simulink model "FINAL"  (R2019a)
settings: Solver=VariableStepAuto  StartTime=0.0  StopTime=5  FixedStep=0.0001  RelTol=1e-3
PreLoadFcn:
  | initDuckWPT
InitFcn:
  | initDuckWPT
StartFcn:
  | initDuckWPT
values from neighbouring files (symbols this model uses):
  angleTolerance = 2    [initDuckWPT.m]
  eeTolerance = 0.01    [initDuckWPT.m]
  JointBounds1 = [-pi/2       pi ... (first row only)    [initDuckWPT.m]
  JointBounds2 = [-pi/3       pi/3 ... (first row only)    [initDuckWPT.m]
  rotM1 = roty(90)*rotx(90)    [initDuckWPT.m]
  trajectory = [0.4  0.4  0.4  0.4  0.4  0.4  0.4 ... (first row only)    [initDuckWPT.m]
undefined symbols (not defined in the file or in its folder): DiscIntNeverNeededParam, X, Y, Z
libraries: sm_lib x205, fl_lib x72, nesl_utility x43, fl_ps_legacy_lib x18, fuzblock x16, Contact_Forces_Lib x12
(part 7 of 7)

== system FINAL/Environment/Robot/Rotational Hardstop51/  1 ==
  External Force and Torque B : sm_lib/Forces and Torques/External Force and Torque  ForceResolutionFrame=AttachedFrame  EnableForceX=off  EnableForceY=off  EnableForceZ=off  EnableForce=off  TorqueResolutionFrame=AttachedFrame  EnableTorqueX=off  EnableTorqueY=off  EnableTorqueZ=on  EnableTorque=off
  External Force and Torque F : sm_lib/Forces and Torques/External Force and Torque  ForceResolutionFrame=AttachedFrame  EnableForceX=off  EnableForceY=off  EnableForceZ=off  EnableForce=off  TorqueResolutionFrame=AttachedFrame  EnableTorqueX=off  EnableTorqueY=off  EnableTorqueZ=on  EnableTorque=off
  Ideal Angular Velocity Source : fl_lib/Mechanical/Mechanical Sources/Ideal Angular Velocity Source
  Ideal Torque Sensor : fl_lib/Mechanical/Mechanical Sensors/Ideal Torque Sensor
  Sign Force B : fl_ps_legacy_lib/Legacy Physical Signals/Functions/PS Gain  gain=-1
      settings: SourceProductName=Simscape
  Transform Sensor : sm_lib/Frames and Transforms/Transform Sensor  MeasurementFrame=Base  SenseAngle=off  SenseAxis=off  SenseAngle1=off  SenseAngle2=off  SenseAngle3=off  SenseQ=off  SenseR=off  SenseOmegaX=off  SenseOmegaY=off  SenseOmegaZ=on  SenseOmega1=off  SenseOmega2=off  SenseOmega3=off  SenseQDot=off  SenseRDot=off  SenseAlphaX=off  SenseAlphaY=off  SenseAlphaZ=off  SenseAlpha1=off  SenseAlpha2=off  SenseAlpha3=off  SenseQDDot=off  SenseRDDot=off  SenseX=off  SenseY=off  SenseZ=off  SenseRad=off  SenseAzim=off  SenseDist=off  SenseInc=off  SenseXDot=off  SenseYDot=off  SenseZDot=off  SenseRadDot=off  SenseAzimDot=off  SenseDistDot=off  SenseIncDot=off  SenseXDDot=off  SenseYDDot=off  SenseZDDot=off  SenseRadDDot=off  SenseAzimDDot=off  SenseDistDDot=off  SenseIncDDot=off
  B : PMIOPort  Side=Left
  F : PMIOPort  Port=2  Side=Right
  R : PMIOPort  Port=3  Side=Right
  C : PMIOPort  Port=4  Side=Left
  connections:
  Ideal Angular Velocity Source/RConn1 -- Transform Sensor/RConn2
  Sign Force B/RConn1 -- External Force and Torque B/LConn1
  B/RConn1 -- External Force and Torque B/RConn1 -- Transform Sensor/LConn1
  External Force and Torque F/RConn1 -- Transform Sensor/RConn1 -- F/RConn1
  C/RConn1 -- Ideal Torque Sensor/RConn1
  External Force and Torque F/LConn1 -- Sign Force B/LConn1 -- Ideal Torque Sensor/RConn2
  Ideal Torque Sensor/LConn1 -- Ideal Angular Velocity Source/RConn2
  R/RConn1 -- Ideal Angular Velocity Source/LConn1

== system FINAL/Environment/Robot/Rotational Hardstop52/  1 ==
  External Force and Torque B : sm_lib/Forces and Torques/External Force and Torque  ForceResolutionFrame=AttachedFrame  EnableForceX=off  EnableForceY=off  EnableForceZ=off  EnableForce=off  TorqueResolutionFrame=AttachedFrame  EnableTorqueX=off  EnableTorqueY=off  EnableTorqueZ=on  EnableTorque=off
  External Force and Torque F : sm_lib/Forces and Torques/External Force and Torque  ForceResolutionFrame=AttachedFrame  EnableForceX=off  EnableForceY=off  EnableForceZ=off  EnableForce=off  TorqueResolutionFrame=AttachedFrame  EnableTorqueX=off  EnableTorqueY=off  EnableTorqueZ=on  EnableTorque=off
  Ideal Angular Velocity Source : fl_lib/Mechanical/Mechanical Sources/Ideal Angular Velocity Source
  Ideal Torque Sensor : fl_lib/Mechanical/Mechanical Sensors/Ideal Torque Sensor
  Sign Force B : fl_ps_legacy_lib/Legacy Physical Signals/Functions/PS Gain  gain=-1
      settings: SourceProductName=Simscape
  Transform Sensor : sm_lib/Frames and Transforms/Transform Sensor  MeasurementFrame=Base  SenseAngle=off  SenseAxis=off  SenseAngle1=off  SenseAngle2=off  SenseAngle3=off  SenseQ=off  SenseR=off  SenseOmegaX=off  SenseOmegaY=off  SenseOmegaZ=on  SenseOmega1=off  SenseOmega2=off  SenseOmega3=off  SenseQDot=off  SenseRDot=off  SenseAlphaX=off  SenseAlphaY=off  SenseAlphaZ=off  SenseAlpha1=off  SenseAlpha2=off  SenseAlpha3=off  SenseQDDot=off  SenseRDDot=off  SenseX=off  SenseY=off  SenseZ=off  SenseRad=off  SenseAzim=off  SenseDist=off  SenseInc=off  SenseXDot=off  SenseYDot=off  SenseZDot=off  SenseRadDot=off  SenseAzimDot=off  SenseDistDot=off  SenseIncDot=off  SenseXDDot=off  SenseYDDot=off  SenseZDDot=off  SenseRadDDot=off  SenseAzimDDot=off  SenseDistDDot=off  SenseIncDDot=off
  B : PMIOPort  Side=Left
  F : PMIOPort  Port=2  Side=Right
  R : PMIOPort  Port=3  Side=Right
  C : PMIOPort  Port=4  Side=Left
  connections:
  R/RConn1 -- Ideal Angular Velocity Source/LConn1
  Ideal Torque Sensor/LConn1 -- Ideal Angular Velocity Source/RConn2
  Ideal Torque Sensor/RConn2 -- Sign Force B/LConn1 -- External Force and Torque F/LConn1
  C/RConn1 -- Ideal Torque Sensor/RConn1
  F/RConn1 -- Transform Sensor/RConn1 -- External Force and Torque F/RConn1
  Transform Sensor/LConn1 -- External Force and Torque B/RConn1 -- B/RConn1
  Sign Force B/RConn1 -- External Force and Torque B/LConn1
  Ideal Angular Velocity Source/RConn1 -- Transform Sensor/RConn2

== system FINAL/Environment/Robot/Rotational Hardstop61/  1 ==
  External Force and Torque B : sm_lib/Forces and Torques/External Force and Torque  ForceResolutionFrame=AttachedFrame  EnableForceX=off  EnableForceY=off  EnableForceZ=off  EnableForce=off  TorqueResolutionFrame=AttachedFrame  EnableTorqueX=off  EnableTorqueY=off  EnableTorqueZ=on  EnableTorque=off
  External Force and Torque F : sm_lib/Forces and Torques/External Force and Torque  ForceResolutionFrame=AttachedFrame  EnableForceX=off  EnableForceY=off  EnableForceZ=off  EnableForce=off  TorqueResolutionFrame=AttachedFrame  EnableTorqueX=off  EnableTorqueY=off  EnableTorqueZ=on  EnableTorque=off
  Ideal Angular Velocity Source : fl_lib/Mechanical/Mechanical Sources/Ideal Angular Velocity Source
  Ideal Torque Sensor : fl_lib/Mechanical/Mechanical Sensors/Ideal Torque Sensor
  Sign Force B : fl_ps_legacy_lib/Legacy Physical Signals/Functions/PS Gain  gain=-1
      settings: SourceProductName=Simscape
  Transform Sensor : sm_lib/Frames and Transforms/Transform Sensor  MeasurementFrame=Base  SenseAngle=off  SenseAxis=off  SenseAngle1=off  SenseAngle2=off  SenseAngle3=off  SenseQ=off  SenseR=off  SenseOmegaX=off  SenseOmegaY=off  SenseOmegaZ=on  SenseOmega1=off  SenseOmega2=off  SenseOmega3=off  SenseQDot=off  SenseRDot=off  SenseAlphaX=off  SenseAlphaY=off  SenseAlphaZ=off  SenseAlpha1=off  SenseAlpha2=off  SenseAlpha3=off  SenseQDDot=off  SenseRDDot=off  SenseX=off  SenseY=off  SenseZ=off  SenseRad=off  SenseAzim=off  SenseDist=off  SenseInc=off  SenseXDot=off  SenseYDot=off  SenseZDot=off  SenseRadDot=off  SenseAzimDot=off  SenseDistDot=off  SenseIncDot=off  SenseXDDot=off  SenseYDDot=off  SenseZDDot=off  SenseRadDDot=off  SenseAzimDDot=off  SenseDistDDot=off  SenseIncDDot=off
  B : PMIOPort  Side=Left
  F : PMIOPort  Port=2  Side=Right
  R : PMIOPort  Port=3  Side=Right
  C : PMIOPort  Port=4  Side=Left
  connections:
  R/RConn1 -- Ideal Angular Velocity Source/LConn1
  Ideal Torque Sensor/LConn1 -- Ideal Angular Velocity Source/RConn2
  Ideal Torque Sensor/RConn2 -- Sign Force B/LConn1 -- External Force and Torque F/LConn1
  C/RConn1 -- Ideal Torque Sensor/RConn1
  F/RConn1 -- Transform Sensor/RConn1 -- External Force and Torque F/RConn1
  Transform Sensor/LConn1 -- External Force and Torque B/RConn1 -- B/RConn1
  Sign Force B/RConn1 -- External Force and Torque B/LConn1
  Ideal Angular Velocity Source/RConn1 -- Transform Sensor/RConn2

== system FINAL/Environment/Robot/Rotational Hardstop62/  1 ==
  External Force and Torque B : sm_lib/Forces and Torques/External Force and Torque  ForceResolutionFrame=AttachedFrame  EnableForceX=off  EnableForceY=off  EnableForceZ=off  EnableForce=off  TorqueResolutionFrame=AttachedFrame  EnableTorqueX=off  EnableTorqueY=off  EnableTorqueZ=on  EnableTorque=off
  External Force and Torque F : sm_lib/Forces and Torques/External Force and Torque  ForceResolutionFrame=AttachedFrame  EnableForceX=off  EnableForceY=off  EnableForceZ=off  EnableForce=off  TorqueResolutionFrame=AttachedFrame  EnableTorqueX=off  EnableTorqueY=off  EnableTorqueZ=on  EnableTorque=off
  Ideal Angular Velocity Source : fl_lib/Mechanical/Mechanical Sources/Ideal Angular Velocity Source
  Ideal Torque Sensor : fl_lib/Mechanical/Mechanical Sensors/Ideal Torque Sensor
  Sign Force B : fl_ps_legacy_lib/Legacy Physical Signals/Functions/PS Gain  gain=-1
      settings: SourceProductName=Simscape
  Transform Sensor : sm_lib/Frames and Transforms/Transform Sensor  MeasurementFrame=Base  SenseAngle=off  SenseAxis=off  SenseAngle1=off  SenseAngle2=off  SenseAngle3=off  SenseQ=off  SenseR=off  SenseOmegaX=off  SenseOmegaY=off  SenseOmegaZ=on  SenseOmega1=off  SenseOmega2=off  SenseOmega3=off  SenseQDot=off  SenseRDot=off  SenseAlphaX=off  SenseAlphaY=off  SenseAlphaZ=off  SenseAlpha1=off  SenseAlpha2=off  SenseAlpha3=off  SenseQDDot=off  SenseRDDot=off  SenseX=off  SenseY=off  SenseZ=off  SenseRad=off  SenseAzim=off  SenseDist=off  SenseInc=off  SenseXDot=off  SenseYDot=off  SenseZDot=off  SenseRadDot=off  SenseAzimDot=off  SenseDistDot=off  SenseIncDot=off  SenseXDDot=off  SenseYDDot=off  SenseZDDot=off  SenseRadDDot=off  SenseAzimDDot=off  SenseDistDDot=off  SenseIncDDot=off
  B : PMIOPort  Side=Left
  F : PMIOPort  Port=2  Side=Right
  R : PMIOPort  Port=3  Side=Right
  C : PMIOPort  Port=4  Side=Left
  connections:
  Ideal Angular Velocity Source/RConn1 -- Transform Sensor/RConn2
  Sign Force B/RConn1 -- External Force and Torque B/LConn1
  B/RConn1 -- External Force and Torque B/RConn1 -- Transform Sensor/LConn1
  External Force and Torque F/RConn1 -- Transform Sensor/RConn1 -- F/RConn1
  C/RConn1 -- Ideal Torque Sensor/RConn1
  External Force and Torque F/LConn1 -- Sign Force B/LConn1 -- Ideal Torque Sensor/RConn2
  Ideal Torque Sensor/LConn1 -- Ideal Angular Velocity Source/RConn2
  R/RConn1 -- Ideal Angular Velocity Source/LConn1

== system FINAL/Environment/Robot/Rotational Hardstop71/  1 ==
  External Force and Torque B : sm_lib/Forces and Torques/External Force and Torque  ForceResolutionFrame=AttachedFrame  EnableForceX=off  EnableForceY=off  EnableForceZ=off  EnableForce=off  TorqueResolutionFrame=AttachedFrame  EnableTorqueX=off  EnableTorqueY=off  EnableTorqueZ=on  EnableTorque=off
  External Force and Torque F : sm_lib/Forces and Torques/External Force and Torque  ForceResolutionFrame=AttachedFrame  EnableForceX=off  EnableForceY=off  EnableForceZ=off  EnableForce=off  TorqueResolutionFrame=AttachedFrame  EnableTorqueX=off  EnableTorqueY=off  EnableTorqueZ=on  EnableTorque=off
  Ideal Angular Velocity Source : fl_lib/Mechanical/Mechanical Sources/Ideal Angular Velocity Source
  Ideal Torque Sensor : fl_lib/Mechanical/Mechanical Sensors/Ideal Torque Sensor
  Sign Force B : fl_ps_legacy_lib/Legacy Physical Signals/Functions/PS Gain  gain=-1
      settings: SourceProductName=Simscape
  Transform Sensor : sm_lib/Frames and Transforms/Transform Sensor  MeasurementFrame=Base  SenseAngle=off  SenseAxis=off  SenseAngle1=off  SenseAngle2=off  SenseAngle3=off  SenseQ=off  SenseR=off  SenseOmegaX=off  SenseOmegaY=off  SenseOmegaZ=on  SenseOmega1=off  SenseOmega2=off  SenseOmega3=off  SenseQDot=off  SenseRDot=off  SenseAlphaX=off  SenseAlphaY=off  SenseAlphaZ=off  SenseAlpha1=off  SenseAlpha2=off  SenseAlpha3=off  SenseQDDot=off  SenseRDDot=off  SenseX=off  SenseY=off  SenseZ=off  SenseRad=off  SenseAzim=off  SenseDist=off  SenseInc=off  SenseXDot=off  SenseYDot=off  SenseZDot=off  SenseRadDot=off  SenseAzimDot=off  SenseDistDot=off  SenseIncDot=off  SenseXDDot=off  SenseYDDot=off  SenseZDDot=off  SenseRadDDot=off  SenseAzimDDot=off  SenseDistDDot=off  SenseIncDDot=off
  B : PMIOPort  Side=Left
  F : PMIOPort  Port=2  Side=Right
  R : PMIOPort  Port=3  Side=Right
  C : PMIOPort  Port=4  Side=Left
  connections:
  Ideal Angular Velocity Source/RConn1 -- Transform Sensor/RConn2
  Sign Force B/RConn1 -- External Force and Torque B/LConn1
  B/RConn1 -- External Force and Torque B/RConn1 -- Transform Sensor/LConn1
  External Force and Torque F/RConn1 -- Transform Sensor/RConn1 -- F/RConn1
  C/RConn1 -- Ideal Torque Sensor/RConn1
  External Force and Torque F/LConn1 -- Sign Force B/LConn1 -- Ideal Torque Sensor/RConn2
  Ideal Torque Sensor/LConn1 -- Ideal Angular Velocity Source/RConn2
  R/RConn1 -- Ideal Angular Velocity Source/LConn1

== system FINAL/Environment/Robot/Rotational Hardstop72/  1 ==
  External Force and Torque B : sm_lib/Forces and Torques/External Force and Torque  ForceResolutionFrame=AttachedFrame  EnableForceX=off  EnableForceY=off  EnableForceZ=off  EnableForce=off  TorqueResolutionFrame=AttachedFrame  EnableTorqueX=off  EnableTorqueY=off  EnableTorqueZ=on  EnableTorque=off
  External Force and Torque F : sm_lib/Forces and Torques/External Force and Torque  ForceResolutionFrame=AttachedFrame  EnableForceX=off  EnableForceY=off  EnableForceZ=off  EnableForce=off  TorqueResolutionFrame=AttachedFrame  EnableTorqueX=off  EnableTorqueY=off  EnableTorqueZ=on  EnableTorque=off
  Ideal Angular Velocity Source : fl_lib/Mechanical/Mechanical Sources/Ideal Angular Velocity Source
  Ideal Torque Sensor : fl_lib/Mechanical/Mechanical Sensors/Ideal Torque Sensor
  Sign Force B : fl_ps_legacy_lib/Legacy Physical Signals/Functions/PS Gain  gain=-1
      settings: SourceProductName=Simscape
  Transform Sensor : sm_lib/Frames and Transforms/Transform Sensor  MeasurementFrame=Base  SenseAngle=off  SenseAxis=off  SenseAngle1=off  SenseAngle2=off  SenseAngle3=off  SenseQ=off  SenseR=off  SenseOmegaX=off  SenseOmegaY=off  SenseOmegaZ=on  SenseOmega1=off  SenseOmega2=off  SenseOmega3=off  SenseQDot=off  SenseRDot=off  SenseAlphaX=off  SenseAlphaY=off  SenseAlphaZ=off  SenseAlpha1=off  SenseAlpha2=off  SenseAlpha3=off  SenseQDDot=off  SenseRDDot=off  SenseX=off  SenseY=off  SenseZ=off  SenseRad=off  SenseAzim=off  SenseDist=off  SenseInc=off  SenseXDot=off  SenseYDot=off  SenseZDot=off  SenseRadDot=off  SenseAzimDot=off  SenseDistDot=off  SenseIncDot=off  SenseXDDot=off  SenseYDDot=off  SenseZDDot=off  SenseRadDDot=off  SenseAzimDDot=off  SenseDistDDot=off  SenseIncDDot=off
  B : PMIOPort  Side=Left
  F : PMIOPort  Port=2  Side=Right
  R : PMIOPort  Port=3  Side=Right
  C : PMIOPort  Port=4  Side=Left
  connections:
  R/RConn1 -- Ideal Angular Velocity Source/LConn1
  Ideal Torque Sensor/LConn1 -- Ideal Angular Velocity Source/RConn2
  Ideal Torque Sensor/RConn2 -- Sign Force B/LConn1 -- External Force and Torque F/LConn1
  C/RConn1 -- Ideal Torque Sensor/RConn1
  F/RConn1 -- Transform Sensor/RConn1 -- External Force and Torque F/RConn1
  Transform Sensor/LConn1 -- External Force and Torque B/RConn1 -- B/RConn1
  Sign Force B/RConn1 -- External Force and Torque B/LConn1
  Ideal Angular Velocity Source/RConn1 -- Transform Sensor/RConn2

== system FINAL/Physical Controller Fuzzy PID/Fuzzy PID Tuning1/Subsystem1/PID ==
  u : Inport
  Kp : Inport  Port=2
  Kd : Inport  Port=3
  Ki : Inport  Port=4
  Discrete-Time Integrator : DiscreteIntegrator  SampleTime=-1  ICPrevOutput=DiscIntNeverNeededParam  ICPrevScaledInput=DiscIntNeverNeededParam
  Discrete-Time Integrator1 : DiscreteIntegrator  SampleTime=-1  ICPrevOutput=DiscIntNeverNeededParam  ICPrevScaledInput=DiscIntNeverNeededParam
  Gain : Gain  Gain=2
  Product : Product
  Product1 : Product
  Product2 : Product
  Sum : Sum  Inputs=|+-
  Sum1 : Sum  Inputs=+++
  Out1 : Outport
  wires:
  Gain/1 -> Sum1/3, Discrete-Time Integrator1/1
  Kp/1 -> Product/2
  u/1 -> Discrete-Time Integrator/1, Product2/1, Product/1
  Kd/1 -> Product2/2
  Product2/1 -> Sum/1
  Discrete-Time Integrator1/1 -> Sum/2
  Sum/1 -> Gain/1
  Product/1 -> Sum1/1
  Sum1/1 -> Out1/1
  Ki/1 -> Product1/2
  Discrete-Time Integrator/1 -> Product1/1
  Product1/1 -> Sum1/2

== system FINAL/Physical Controller Fuzzy PID/Fuzzy PID Tuning1/Subsystem2/PID ==
  u : Inport
  Kp : Inport  Port=2
  Kd : Inport  Port=3
  Ki : Inport  Port=4
  Discrete-Time Integrator : DiscreteIntegrator  SampleTime=-1  ICPrevOutput=DiscIntNeverNeededParam  ICPrevScaledInput=DiscIntNeverNeededParam
  Discrete-Time Integrator1 : DiscreteIntegrator  SampleTime=-1  ICPrevOutput=DiscIntNeverNeededParam  ICPrevScaledInput=DiscIntNeverNeededParam
  Gain : Gain  Gain=2
  Product : Product
  Product1 : Product
  Product2 : Product
  Sum : Sum  Inputs=|+-
  Sum1 : Sum  Inputs=+++
  Out1 : Outport
  wires:
  Product1/1 -> Sum1/2
  Discrete-Time Integrator/1 -> Product1/1
  Ki/1 -> Product1/2
  Sum1/1 -> Out1/1
  Product/1 -> Sum1/1
  Sum/1 -> Gain/1
  Discrete-Time Integrator1/1 -> Sum/2
  Product2/1 -> Sum/1
  Kd/1 -> Product2/2
  u/1 -> Product/1, Product2/1, Discrete-Time Integrator/1
  Kp/1 -> Product/2
  Gain/1 -> Discrete-Time Integrator1/1, Sum1/3

== system FINAL/Physical Controller Fuzzy PID/Fuzzy PID Tuning1/Subsystem3/PID ==
  u : Inport
  Kp : Inport  Port=2
  Kd : Inport  Port=3
  Ki : Inport  Port=4
  Discrete-Time Integrator : DiscreteIntegrator  SampleTime=-1  ICPrevOutput=DiscIntNeverNeededParam  ICPrevScaledInput=DiscIntNeverNeededParam
  Discrete-Time Integrator1 : DiscreteIntegrator  SampleTime=-1  ICPrevOutput=DiscIntNeverNeededParam  ICPrevScaledInput=DiscIntNeverNeededParam
  Gain : Gain  Gain=2
  Product : Product
  Product1 : Product
  Product2 : Product
  Sum : Sum  Inputs=|+-
  Sum1 : Sum  Inputs=+++
  Out1 : Outport
  wires:
  Product1/1 -> Sum1/2
  Discrete-Time Integrator/1 -> Product1/1
  Ki/1 -> Product1/2
  Sum1/1 -> Out1/1
  Product/1 -> Sum1/1
  Sum/1 -> Gain/1
  Discrete-Time Integrator1/1 -> Sum/2
  Product2/1 -> Sum/1
  Kd/1 -> Product2/2
  u/1 -> Product/1, Product2/1, Discrete-Time Integrator/1
  Kp/1 -> Product/2
  Gain/1 -> Discrete-Time Integrator1/1, Sum1/3

== system FINAL/Physical Controller Fuzzy PID/Fuzzy PID Tuning1/Subsystem4/PID ==
  u : Inport
  Kp : Inport  Port=2
  Kd : Inport  Port=3
  Ki : Inport  Port=4
  Discrete-Time Integrator : DiscreteIntegrator  SampleTime=-1  ICPrevOutput=DiscIntNeverNeededParam  ICPrevScaledInput=DiscIntNeverNeededParam
  Discrete-Time Integrator1 : DiscreteIntegrator  SampleTime=-1  ICPrevOutput=DiscIntNeverNeededParam  ICPrevScaledInput=DiscIntNeverNeededParam
  Gain : Gain  Gain=2
  Product : Product
  Product1 : Product
  Product2 : Product
  Sum : Sum  Inputs=|+-
  Sum1 : Sum  Inputs=+++
  Out1 : Outport
  wires:
  Gain/1 -> Sum1/3, Discrete-Time Integrator1/1
  Kp/1 -> Product/2
  u/1 -> Discrete-Time Integrator/1, Product2/1, Product/1
  Kd/1 -> Product2/2
  Product2/1 -> Sum/1
  Discrete-Time Integrator1/1 -> Sum/2
  Sum/1 -> Gain/1
  Product/1 -> Sum1/1
  Sum1/1 -> Out1/1
  Ki/1 -> Product1/2
  Discrete-Time Integrator/1 -> Product1/1
  Product1/1 -> Sum1/2

== system FINAL/Physical Controller Fuzzy PID/Fuzzy PID Tuning1/Subsystem5/PID ==
  u : Inport
  Kp : Inport  Port=2
  Kd : Inport  Port=3
  Ki : Inport  Port=4
  Discrete-Time Integrator : DiscreteIntegrator  SampleTime=-1  ICPrevOutput=DiscIntNeverNeededParam  ICPrevScaledInput=DiscIntNeverNeededParam
  Discrete-Time Integrator1 : DiscreteIntegrator  SampleTime=-1  ICPrevOutput=DiscIntNeverNeededParam  ICPrevScaledInput=DiscIntNeverNeededParam
  Gain : Gain  Gain=2
  Product : Product
  Product1 : Product
  Product2 : Product
  Sum : Sum  Inputs=|+-
  Sum1 : Sum  Inputs=+++
  Out1 : Outport
  wires:
  Product1/1 -> Sum1/2
  Discrete-Time Integrator/1 -> Product1/1
  Ki/1 -> Product1/2
  Sum1/1 -> Out1/1
  Product/1 -> Sum1/1
  Sum/1 -> Gain/1
  Discrete-Time Integrator1/1 -> Sum/2
  Product2/1 -> Sum/1
  Kd/1 -> Product2/2
  u/1 -> Product/1, Product2/1, Discrete-Time Integrator/1
  Kp/1 -> Product/2
  Gain/1 -> Discrete-Time Integrator1/1, Sum1/3

== system FINAL/Physical Controller Fuzzy PID/Fuzzy PID Tuning1/Subsystem6/PID ==
  u : Inport
  Kp : Inport  Port=2
  Kd : Inport  Port=3
  Ki : Inport  Port=4
  Discrete-Time Integrator : DiscreteIntegrator  SampleTime=-1  ICPrevOutput=DiscIntNeverNeededParam  ICPrevScaledInput=DiscIntNeverNeededParam
  Discrete-Time Integrator1 : DiscreteIntegrator  SampleTime=-1  ICPrevOutput=DiscIntNeverNeededParam  ICPrevScaledInput=DiscIntNeverNeededParam
  Gain : Gain  Gain=2
  Product : Product
  Product1 : Product
  Product2 : Product
  Sum : Sum  Inputs=|+-
  Sum1 : Sum  Inputs=+++
  Out1 : Outport
  wires:
  Gain/1 -> Sum1/3, Discrete-Time Integrator1/1
  Kp/1 -> Product/2
  u/1 -> Discrete-Time Integrator/1, Product2/1, Product/1
  Kd/1 -> Product2/2
  Product2/1 -> Sum/1
  Discrete-Time Integrator1/1 -> Sum/2
  Sum/1 -> Gain/1
  Product/1 -> Sum1/1
  Sum1/1 -> Out1/1
  Ki/1 -> Product1/2
  Discrete-Time Integrator/1 -> Product1/1
  Product1/1 -> Sum1/2

== system FINAL/Physical Controller Fuzzy PID/Fuzzy PID Tuning1/Subsystem7/PID ==
  u : Inport
  Kp : Inport  Port=2
  Kd : Inport  Port=3
  Ki : Inport  Port=4
  Discrete-Time Integrator : DiscreteIntegrator  SampleTime=-1  ICPrevOutput=DiscIntNeverNeededParam  ICPrevScaledInput=DiscIntNeverNeededParam
  Discrete-Time Integrator1 : DiscreteIntegrator  SampleTime=-1  ICPrevOutput=DiscIntNeverNeededParam  ICPrevScaledInput=DiscIntNeverNeededParam
  Gain : Gain  Gain=2
  Product : Product
  Product1 : Product
  Product2 : Product
  Sum : Sum  Inputs=|+-
  Sum1 : Sum  Inputs=+++
  Out1 : Outport
  wires:
  Gain/1 -> Sum1/3, Discrete-Time Integrator1/1
  Kp/1 -> Product/2
  u/1 -> Discrete-Time Integrator/1, Product2/1, Product/1
  Kd/1 -> Product2/2
  Product2/1 -> Sum/1
  Discrete-Time Integrator1/1 -> Sum/2
  Sum/1 -> Gain/1
  Product/1 -> Sum1/1
  Sum1/1 -> Out1/1
  Ki/1 -> Product1/2
  Discrete-Time Integrator/1 -> Product1/1
  Product1/1 -> Sum1/2

== system FINAL/Physical Controller Fuzzy PID/Fuzzy PID Tuning1/Subsystem8/PID ==
  u : Inport
  Kp : Inport  Port=2
  Kd : Inport  Port=3
  Ki : Inport  Port=4
  Discrete-Time Integrator : DiscreteIntegrator  SampleTime=-1  ICPrevOutput=DiscIntNeverNeededParam  ICPrevScaledInput=DiscIntNeverNeededParam
  Discrete-Time Integrator1 : DiscreteIntegrator  SampleTime=-1  ICPrevOutput=DiscIntNeverNeededParam  ICPrevScaledInput=DiscIntNeverNeededParam
  Gain : Gain  Gain=2
  Product : Product
  Product1 : Product
  Product2 : Product
  Sum : Sum  Inputs=|+-
  Sum1 : Sum  Inputs=+++
  Out1 : Outport
  wires:
  Product1/1 -> Sum1/2
  Discrete-Time Integrator/1 -> Product1/1
  Ki/1 -> Product1/2
  Sum1/1 -> Out1/1
  Product/1 -> Sum1/1
  Sum/1 -> Gain/1
  Discrete-Time Integrator1/1 -> Sum/2
  Product2/1 -> Sum/1
  Kd/1 -> Product2/2
  u/1 -> Product/1, Product2/1, Discrete-Time Integrator/1
  Kp/1 -> Product/2
  Gain/1 -> Discrete-Time Integrator1/1, Sum1/3

== system FINAL/Physical Controller Fuzzy PID/Fuzzy PID Tuning2/Subsystem1/PID ==
  u : Inport
  Kp : Inport  Port=2
  Kd : Inport  Port=3
  Ki : Inport  Port=4
  Discrete-Time Integrator : DiscreteIntegrator  SampleTime=-1  ICPrevOutput=DiscIntNeverNeededParam  ICPrevScaledInput=DiscIntNeverNeededParam
  Discrete-Time Integrator1 : DiscreteIntegrator  SampleTime=-1  ICPrevOutput=DiscIntNeverNeededParam  ICPrevScaledInput=DiscIntNeverNeededParam
  Gain : Gain  Gain=2
  Product : Product
  Product1 : Product
  Product2 : Product
  Sum : Sum  Inputs=|+-
  Sum1 : Sum  Inputs=+++
  Out1 : Outport
  wires:
  Product1/1 -> Sum1/2
  Discrete-Time Integrator/1 -> Product1/1
  Ki/1 -> Product1/2
  Sum1/1 -> Out1/1
  Product/1 -> Sum1/1
  Sum/1 -> Gain/1
  Discrete-Time Integrator1/1 -> Sum/2
  Product2/1 -> Sum/1
  Kd/1 -> Product2/2
  u/1 -> Product/1, Product2/1, Discrete-Time Integrator/1
  Kp/1 -> Product/2
  Gain/1 -> Discrete-Time Integrator1/1, Sum1/3

== system FINAL/Physical Controller Fuzzy PID/Fuzzy PID Tuning2/Subsystem2/PID ==
  u : Inport
  Kp : Inport  Port=2
  Kd : Inport  Port=3
  Ki : Inport  Port=4
  Discrete-Time Integrator : DiscreteIntegrator  SampleTime=-1  ICPrevOutput=DiscIntNeverNeededParam  ICPrevScaledInput=DiscIntNeverNeededParam
  Discrete-Time Integrator1 : DiscreteIntegrator  SampleTime=-1  ICPrevOutput=DiscIntNeverNeededParam  ICPrevScaledInput=DiscIntNeverNeededParam
  Gain : Gain  Gain=2
  Product : Product
  Product1 : Product
  Product2 : Product
  Sum : Sum  Inputs=|+-
  Sum1 : Sum  Inputs=+++
  Out1 : Outport
  wires:
  Gain/1 -> Sum1/3, Discrete-Time Integrator1/1
  Kp/1 -> Product/2
  u/1 -> Discrete-Time Integrator/1, Product2/1, Product/1
  Kd/1 -> Product2/2
  Product2/1 -> Sum/1
  Discrete-Time Integrator1/1 -> Sum/2
  Sum/1 -> Gain/1
  Product/1 -> Sum1/1
  Sum1/1 -> Out1/1
  Ki/1 -> Product1/2
  Discrete-Time Integrator/1 -> Product1/1
  Product1/1 -> Sum1/2

== system FINAL/Physical Controller Fuzzy PID/Fuzzy PID Tuning2/Subsystem3/PID ==
  u : Inport
  Kp : Inport  Port=2
  Kd : Inport  Port=3
  Ki : Inport  Port=4
  Discrete-Time Integrator : DiscreteIntegrator  SampleTime=-1  ICPrevOutput=DiscIntNeverNeededParam  ICPrevScaledInput=DiscIntNeverNeededParam
  Discrete-Time Integrator1 : DiscreteIntegrator  SampleTime=-1  ICPrevOutput=DiscIntNeverNeededParam  ICPrevScaledInput=DiscIntNeverNeededParam
  Gain : Gain  Gain=2
  Product : Product
  Product1 : Product
  Product2 : Product
  Sum : Sum  Inputs=|+-
  Sum1 : Sum  Inputs=+++
  Out1 : Outport
  wires:
  Gain/1 -> Sum1/3, Discrete-Time Integrator1/1
  Kp/1 -> Product/2
  u/1 -> Discrete-Time Integrator/1, Product2/1, Product/1
  Kd/1 -> Product2/2
  Product2/1 -> Sum/1
  Discrete-Time Integrator1/1 -> Sum/2
  Sum/1 -> Gain/1
  Product/1 -> Sum1/1
  Sum1/1 -> Out1/1
  Ki/1 -> Product1/2
  Discrete-Time Integrator/1 -> Product1/1
  Product1/1 -> Sum1/2

== system FINAL/Physical Controller Fuzzy PID/Fuzzy PID Tuning2/Subsystem4/PID ==
  u : Inport
  Kp : Inport  Port=2
  Kd : Inport  Port=3
  Ki : Inport  Port=4
  Discrete-Time Integrator : DiscreteIntegrator  SampleTime=-1  ICPrevOutput=DiscIntNeverNeededParam  ICPrevScaledInput=DiscIntNeverNeededParam
  Discrete-Time Integrator1 : DiscreteIntegrator  SampleTime=-1  ICPrevOutput=DiscIntNeverNeededParam  ICPrevScaledInput=DiscIntNeverNeededParam
  Gain : Gain  Gain=2
  Product : Product
  Product1 : Product
  Product2 : Product
  Sum : Sum  Inputs=|+-
  Sum1 : Sum  Inputs=+++
  Out1 : Outport
  wires:
  Product1/1 -> Sum1/2
  Discrete-Time Integrator/1 -> Product1/1
  Ki/1 -> Product1/2
  Sum1/1 -> Out1/1
  Product/1 -> Sum1/1
  Sum/1 -> Gain/1
  Discrete-Time Integrator1/1 -> Sum/2
  Product2/1 -> Sum/1
  Kd/1 -> Product2/2
  u/1 -> Product/1, Product2/1, Discrete-Time Integrator/1
  Kp/1 -> Product/2
  Gain/1 -> Discrete-Time Integrator1/1, Sum1/3

== system FINAL/Physical Controller Fuzzy PID/Fuzzy PID Tuning2/Subsystem5/PID ==
  u : Inport
  Kp : Inport  Port=2
  Kd : Inport  Port=3
  Ki : Inport  Port=4
  Discrete-Time Integrator : DiscreteIntegrator  SampleTime=-1  ICPrevOutput=DiscIntNeverNeededParam  ICPrevScaledInput=DiscIntNeverNeededParam
  Discrete-Time Integrator1 : DiscreteIntegrator  SampleTime=-1  ICPrevOutput=DiscIntNeverNeededParam  ICPrevScaledInput=DiscIntNeverNeededParam
  Gain : Gain  Gain=2
  Product : Product
  Product1 : Product
  Product2 : Product
  Sum : Sum  Inputs=|+-
  Sum1 : Sum  Inputs=+++
  Out1 : Outport
  wires:
  Gain/1 -> Sum1/3, Discrete-Time Integrator1/1
  Kp/1 -> Product/2
  u/1 -> Discrete-Time Integrator/1, Product2/1, Product/1
  Kd/1 -> Product2/2
  Product2/1 -> Sum/1
  Discrete-Time Integrator1/1 -> Sum/2
  Sum/1 -> Gain/1
  Product/1 -> Sum1/1
  Sum1/1 -> Out1/1
  Ki/1 -> Product1/2
  Discrete-Time Integrator/1 -> Product1/1
  Product1/1 -> Sum1/2

== system FINAL/Physical Controller Fuzzy PID/Fuzzy PID Tuning2/Subsystem6/PID ==
  u : Inport
  Kp : Inport  Port=2
  Kd : Inport  Port=3
  Ki : Inport  Port=4
  Discrete-Time Integrator : DiscreteIntegrator  SampleTime=-1  ICPrevOutput=DiscIntNeverNeededParam  ICPrevScaledInput=DiscIntNeverNeededParam
  Discrete-Time Integrator1 : DiscreteIntegrator  SampleTime=-1  ICPrevOutput=DiscIntNeverNeededParam  ICPrevScaledInput=DiscIntNeverNeededParam
  Gain : Gain  Gain=2
  Product : Product
  Product1 : Product
  Product2 : Product
  Sum : Sum  Inputs=|+-
  Sum1 : Sum  Inputs=+++
  Out1 : Outport
  wires:
  Product1/1 -> Sum1/2
  Discrete-Time Integrator/1 -> Product1/1
  Ki/1 -> Product1/2
  Sum1/1 -> Out1/1
  Product/1 -> Sum1/1
  Sum/1 -> Gain/1
  Discrete-Time Integrator1/1 -> Sum/2
  Product2/1 -> Sum/1
  Kd/1 -> Product2/2
  u/1 -> Product/1, Product2/1, Discrete-Time Integrator/1
  Kp/1 -> Product/2
  Gain/1 -> Discrete-Time Integrator1/1, Sum1/3

== system FINAL/Physical Controller Fuzzy PID/Fuzzy PID Tuning2/Subsystem7/PID ==
  u : Inport
  Kp : Inport  Port=2
  Kd : Inport  Port=3
  Ki : Inport  Port=4
  Discrete-Time Integrator : DiscreteIntegrator  SampleTime=-1  ICPrevOutput=DiscIntNeverNeededParam  ICPrevScaledInput=DiscIntNeverNeededParam
  Discrete-Time Integrator1 : DiscreteIntegrator  SampleTime=-1  ICPrevOutput=DiscIntNeverNeededParam  ICPrevScaledInput=DiscIntNeverNeededParam
  Gain : Gain  Gain=2
  Product : Product
  Product1 : Product
  Product2 : Product
  Sum : Sum  Inputs=|+-
  Sum1 : Sum  Inputs=+++
  Out1 : Outport
  wires:
  Product1/1 -> Sum1/2
  Discrete-Time Integrator/1 -> Product1/1
  Ki/1 -> Product1/2
  Sum1/1 -> Out1/1
  Product/1 -> Sum1/1
  Sum/1 -> Gain/1
  Discrete-Time Integrator1/1 -> Sum/2
  Product2/1 -> Sum/1
  Kd/1 -> Product2/2
  u/1 -> Product/1, Product2/1, Discrete-Time Integrator/1
  Kp/1 -> Product/2
  Gain/1 -> Discrete-Time Integrator1/1, Sum1/3

== system FINAL/Physical Controller Fuzzy PID/Fuzzy PID Tuning2/Subsystem8/PID ==
  u : Inport
  Kp : Inport  Port=2
  Kd : Inport  Port=3
  Ki : Inport  Port=4
  Discrete-Time Integrator : DiscreteIntegrator  SampleTime=-1  ICPrevOutput=DiscIntNeverNeededParam  ICPrevScaledInput=DiscIntNeverNeededParam
  Discrete-Time Integrator1 : DiscreteIntegrator  SampleTime=-1  ICPrevOutput=DiscIntNeverNeededParam  ICPrevScaledInput=DiscIntNeverNeededParam
  Gain : Gain  Gain=2
  Product : Product
  Product1 : Product
  Product2 : Product
  Sum : Sum  Inputs=|+-
  Sum1 : Sum  Inputs=+++
  Out1 : Outport
  wires:
  Gain/1 -> Sum1/3, Discrete-Time Integrator1/1
  Kp/1 -> Product/2
  u/1 -> Discrete-Time Integrator/1, Product2/1, Product/1
  Kd/1 -> Product2/2
  Product2/1 -> Sum/1
  Discrete-Time Integrator1/1 -> Sum/2
  Sum/1 -> Gain/1
  Product/1 -> Sum1/1
  Sum1/1 -> Out1/1
  Ki/1 -> Product1/2
  Discrete-Time Integrator/1 -> Product1/1
  Product1/1 -> Sum1/2

== system FINAL/Environment/Robot/Hand1/Rotational Hardstop/  1 ==
  External Force and Torque B : sm_lib/Forces and Torques/External Force and Torque  ForceResolutionFrame=AttachedFrame  EnableForceX=off  EnableForceY=off  EnableForceZ=off  EnableForce=off  TorqueResolutionFrame=AttachedFrame  EnableTorqueX=off  EnableTorqueY=off  EnableTorqueZ=on  EnableTorque=off
  External Force and Torque F : sm_lib/Forces and Torques/External Force and Torque  ForceResolutionFrame=AttachedFrame  EnableForceX=off  EnableForceY=off  EnableForceZ=off  EnableForce=off  TorqueResolutionFrame=AttachedFrame  EnableTorqueX=off  EnableTorqueY=off  EnableTorqueZ=on  EnableTorque=off
  Ideal Angular Velocity Source : fl_lib/Mechanical/Mechanical Sources/Ideal Angular Velocity Source
  Ideal Torque Sensor : fl_lib/Mechanical/Mechanical Sensors/Ideal Torque Sensor
  Sign Force B : fl_ps_legacy_lib/Legacy Physical Signals/Functions/PS Gain  gain=-1
      settings: SourceProductName=Simscape
  Transform Sensor : sm_lib/Frames and Transforms/Transform Sensor  MeasurementFrame=Base  SenseAngle=off  SenseAxis=off  SenseAngle1=off  SenseAngle2=off  SenseAngle3=off  SenseQ=off  SenseR=off  SenseOmegaX=off  SenseOmegaY=off  SenseOmegaZ=on  SenseOmega1=off  SenseOmega2=off  SenseOmega3=off  SenseQDot=off  SenseRDot=off  SenseAlphaX=off  SenseAlphaY=off  SenseAlphaZ=off  SenseAlpha1=off  SenseAlpha2=off  SenseAlpha3=off  SenseQDDot=off  SenseRDDot=off  SenseX=off  SenseY=off  SenseZ=off  SenseRad=off  SenseAzim=off  SenseDist=off  SenseInc=off  SenseXDot=off  SenseYDot=off  SenseZDot=off  SenseRadDot=off  SenseAzimDot=off  SenseDistDot=off  SenseIncDot=off  SenseXDDot=off  SenseYDDot=off  SenseZDDot=off  SenseRadDDot=off  SenseAzimDDot=off  SenseDistDDot=off  SenseIncDDot=off
  B : PMIOPort  Side=Left
  F : PMIOPort  Port=2  Side=Right
  R : PMIOPort  Port=3  Side=Right
  C : PMIOPort  Port=4  Side=Left
  connections:
  Ideal Angular Velocity Source/RConn1 -- Transform Sensor/RConn2
  Sign Force B/RConn1 -- External Force and Torque B/LConn1
  B/RConn1 -- External Force and Torque B/RConn1 -- Transform Sensor/LConn1
  External Force and Torque F/RConn1 -- Transform Sensor/RConn1 -- F/RConn1
  C/RConn1 -- Ideal Torque Sensor/RConn1
  External Force and Torque F/LConn1 -- Sign Force B/LConn1 -- Ideal Torque Sensor/RConn2
  Ideal Torque Sensor/LConn1 -- Ideal Angular Velocity Source/RConn2
  R/RConn1 -- Ideal Angular Velocity Source/LConn1

== system FINAL/Environment/Robot/Hand1/Rotational Hardstop1/  1 ==
  External Force and Torque B : sm_lib/Forces and Torques/External Force and Torque  ForceResolutionFrame=AttachedFrame  EnableForceX=off  EnableForceY=off  EnableForceZ=off  EnableForce=off  TorqueResolutionFrame=AttachedFrame  EnableTorqueX=off  EnableTorqueY=off  EnableTorqueZ=on  EnableTorque=off
  External Force and Torque F : sm_lib/Forces and Torques/External Force and Torque  ForceResolutionFrame=AttachedFrame  EnableForceX=off  EnableForceY=off  EnableForceZ=off  EnableForce=off  TorqueResolutionFrame=AttachedFrame  EnableTorqueX=off  EnableTorqueY=off  EnableTorqueZ=on  EnableTorque=off
  Ideal Angular Velocity Source : fl_lib/Mechanical/Mechanical Sources/Ideal Angular Velocity Source
  Ideal Torque Sensor : fl_lib/Mechanical/Mechanical Sensors/Ideal Torque Sensor
  Sign Force B : fl_ps_legacy_lib/Legacy Physical Signals/Functions/PS Gain  gain=-1
      settings: SourceProductName=Simscape
  Transform Sensor : sm_lib/Frames and Transforms/Transform Sensor  MeasurementFrame=Base  SenseAngle=off  SenseAxis=off  SenseAngle1=off  SenseAngle2=off  SenseAngle3=off  SenseQ=off  SenseR=off  SenseOmegaX=off  SenseOmegaY=off  SenseOmegaZ=on  SenseOmega1=off  SenseOmega2=off  SenseOmega3=off  SenseQDot=off  SenseRDot=off  SenseAlphaX=off  SenseAlphaY=off  SenseAlphaZ=off  SenseAlpha1=off  SenseAlpha2=off  SenseAlpha3=off  SenseQDDot=off  SenseRDDot=off  SenseX=off  SenseY=off  SenseZ=off  SenseRad=off  SenseAzim=off  SenseDist=off  SenseInc=off  SenseXDot=off  SenseYDot=off  SenseZDot=off  SenseRadDot=off  SenseAzimDot=off  SenseDistDot=off  SenseIncDot=off  SenseXDDot=off  SenseYDDot=off  SenseZDDot=off  SenseRadDDot=off  SenseAzimDDot=off  SenseDistDDot=off  SenseIncDDot=off
  B : PMIOPort  Side=Left
  F : PMIOPort  Port=2  Side=Right
  R : PMIOPort  Port=3  Side=Right
  C : PMIOPort  Port=4  Side=Left
  connections:
  R/RConn1 -- Ideal Angular Velocity Source/LConn1
  Ideal Torque Sensor/LConn1 -- Ideal Angular Velocity Source/RConn2
  Ideal Torque Sensor/RConn2 -- Sign Force B/LConn1 -- External Force and Torque F/LConn1
  C/RConn1 -- Ideal Torque Sensor/RConn1
  F/RConn1 -- Transform Sensor/RConn1 -- External Force and Torque F/RConn1
  Transform Sensor/LConn1 -- External Force and Torque B/RConn1 -- B/RConn1
  Sign Force B/RConn1 -- External Force and Torque B/LConn1
  Ideal Angular Velocity Source/RConn1 -- Transform Sensor/RConn2

== system FINAL/Environment/Robot/Hand2/Rotational Hardstop/  1 ==
  External Force and Torque B : sm_lib/Forces and Torques/External Force and Torque  ForceResolutionFrame=AttachedFrame  EnableForceX=off  EnableForceY=off  EnableForceZ=off  EnableForce=off  TorqueResolutionFrame=AttachedFrame  EnableTorqueX=off  EnableTorqueY=off  EnableTorqueZ=on  EnableTorque=off
  External Force and Torque F : sm_lib/Forces and Torques/External Force and Torque  ForceResolutionFrame=AttachedFrame  EnableForceX=off  EnableForceY=off  EnableForceZ=off  EnableForce=off  TorqueResolutionFrame=AttachedFrame  EnableTorqueX=off  EnableTorqueY=off  EnableTorqueZ=on  EnableTorque=off
  Ideal Angular Velocity Source : fl_lib/Mechanical/Mechanical Sources/Ideal Angular Velocity Source
  Ideal Torque Sensor : fl_lib/Mechanical/Mechanical Sensors/Ideal Torque Sensor
  Sign Force B : fl_ps_legacy_lib/Legacy Physical Signals/Functions/PS Gain  gain=-1
      settings: SourceProductName=Simscape
  Transform Sensor : sm_lib/Frames and Transforms/Transform Sensor  MeasurementFrame=Base  SenseAngle=off  SenseAxis=off  SenseAngle1=off  SenseAngle2=off  SenseAngle3=off  SenseQ=off  SenseR=off  SenseOmegaX=off  SenseOmegaY=off  SenseOmegaZ=on  SenseOmega1=off  SenseOmega2=off  SenseOmega3=off  SenseQDot=off  SenseRDot=off  SenseAlphaX=off  SenseAlphaY=off  SenseAlphaZ=off  SenseAlpha1=off  SenseAlpha2=off  SenseAlpha3=off  SenseQDDot=off  SenseRDDot=off  SenseX=off  SenseY=off  SenseZ=off  SenseRad=off  SenseAzim=off  SenseDist=off  SenseInc=off  SenseXDot=off  SenseYDot=off  SenseZDot=off  SenseRadDot=off  SenseAzimDot=off  SenseDistDot=off  SenseIncDot=off  SenseXDDot=off  SenseYDDot=off  SenseZDDot=off  SenseRadDDot=off  SenseAzimDDot=off  SenseDistDDot=off  SenseIncDDot=off
  B : PMIOPort  Side=Left
  F : PMIOPort  Port=2  Side=Right
  R : PMIOPort  Port=3  Side=Right
  C : PMIOPort  Port=4  Side=Left
  connections:
  Ideal Angular Velocity Source/RConn1 -- Transform Sensor/RConn2
  Sign Force B/RConn1 -- External Force and Torque B/LConn1
  B/RConn1 -- External Force and Torque B/RConn1 -- Transform Sensor/LConn1
  External Force and Torque F/RConn1 -- Transform Sensor/RConn1 -- F/RConn1
  C/RConn1 -- Ideal Torque Sensor/RConn1
  External Force and Torque F/LConn1 -- Sign Force B/LConn1 -- Ideal Torque Sensor/RConn2
  Ideal Torque Sensor/LConn1 -- Ideal Angular Velocity Source/RConn2
  R/RConn1 -- Ideal Angular Velocity Source/LConn1

== system FINAL/Environment/Robot/Hand2/Rotational Hardstop1/  1 ==
  External Force and Torque B : sm_lib/Forces and Torques/External Force and Torque  ForceResolutionFrame=AttachedFrame  EnableForceX=off  EnableForceY=off  EnableForceZ=off  EnableForce=off  TorqueResolutionFrame=AttachedFrame  EnableTorqueX=off  EnableTorqueY=off  EnableTorqueZ=on  EnableTorque=off
  External Force and Torque F : sm_lib/Forces and Torques/External Force and Torque  ForceResolutionFrame=AttachedFrame  EnableForceX=off  EnableForceY=off  EnableForceZ=off  EnableForce=off  TorqueResolutionFrame=AttachedFrame  EnableTorqueX=off  EnableTorqueY=off  EnableTorqueZ=on  EnableTorque=off
  Ideal Angular Velocity Source : fl_lib/Mechanical/Mechanical Sources/Ideal Angular Velocity Source
  Ideal Torque Sensor : fl_lib/Mechanical/Mechanical Sensors/Ideal Torque Sensor
  Sign Force B : fl_ps_legacy_lib/Legacy Physical Signals/Functions/PS Gain  gain=-1
      settings: SourceProductName=Simscape
  Transform Sensor : sm_lib/Frames and Transforms/Transform Sensor  MeasurementFrame=Base  SenseAngle=off  SenseAxis=off  SenseAngle1=off  SenseAngle2=off  SenseAngle3=off  SenseQ=off  SenseR=off  SenseOmegaX=off  SenseOmegaY=off  SenseOmegaZ=on  SenseOmega1=off  SenseOmega2=off  SenseOmega3=off  SenseQDot=off  SenseRDot=off  SenseAlphaX=off  SenseAlphaY=off  SenseAlphaZ=off  SenseAlpha1=off  SenseAlpha2=off  SenseAlpha3=off  SenseQDDot=off  SenseRDDot=off  SenseX=off  SenseY=off  SenseZ=off  SenseRad=off  SenseAzim=off  SenseDist=off  SenseInc=off  SenseXDot=off  SenseYDot=off  SenseZDot=off  SenseRadDot=off  SenseAzimDot=off  SenseDistDot=off  SenseIncDot=off  SenseXDDot=off  SenseYDDot=off  SenseZDDot=off  SenseRadDDot=off  SenseAzimDDot=off  SenseDistDDot=off  SenseIncDDot=off
  B : PMIOPort  Side=Left
  F : PMIOPort  Port=2  Side=Right
  R : PMIOPort  Port=3  Side=Right
  C : PMIOPort  Port=4  Side=Left
  connections:
  R/RConn1 -- Ideal Angular Velocity Source/LConn1
  Ideal Torque Sensor/LConn1 -- Ideal Angular Velocity Source/RConn2
  Ideal Torque Sensor/RConn2 -- Sign Force B/LConn1 -- External Force and Torque F/LConn1
  C/RConn1 -- Ideal Torque Sensor/RConn1
  F/RConn1 -- Transform Sensor/RConn1 -- External Force and Torque F/RConn1
  Transform Sensor/LConn1 -- External Force and Torque B/RConn1 -- B/RConn1
  Sign Force B/RConn1 -- External Force and Torque B/LConn1
  Ideal Angular Velocity Source/RConn1 -- Transform Sensor/RConn2

== stateflow chart FINAL/Supervisory Controller & Inverse Kinematics BOTH ARMS/BOTH ARMS SUPERVISORY CONTROLLER & INVERSE KINEMATICS ==
  state GRABBING
    entry:
    ReachedState=2;
    entry,during:
    GripCommand=1;
    PosDiffR=eePoseR-TargetPosR;
    PosDiffL=eePoseL-TargetPosL;
  state DETECTION_AND_OBJECT_APPROACH
    entry:
    ReachedState=1;
    TargetPosR=ObjectPosition+[0;-0.26;0.025];
    TargetPosL=ObjectPosition+[0;0.26;0.025];
    DesiredJointStatesR=GenInvKinR(PreviousMeasureR,TargetPosR,rotM1,JointBounds1);
    DesiredJointStatesL=DesiredJointStatesR;
    entry,during:
    GripCommand=0;
    PosDiffR=eePoseR-TargetPosR;
    PosDiffL=eePoseL-TargetPosL;
    AngleRef=90;
  state ENDING
    entry:
    ReachedState=ReachedState+1;
    entry,during:
    GripCommand=0;
    PosDiffR=[0;0;0];
    PosDiffL=[0;0;0];
  state WAIT_GRABBING
    entry,during:
    GripCommand=1;
    PosDiffR=eePoseR-TargetPosR;
    PosDiffL=eePoseL-TargetPosL;
  state DELAY_CHECKING
    entry,during:
    GripCommand=1;
    PosDiffR=eePoseR-TargetPosR;
    PosDiffL=eePoseL-TargetPosL;
  state SET_CONFIG
    entry:
    ReachedState=ReachedState+1;
    CurrentState=CurrentState+1;
    TargetPosR=Trajectory(1:3,CurrentState)+0.27*[0;-cos(Trajectory(4,CurrentState)/180*pi);-sin(Trajectory(4,CurrentState)/180*pi)];
    TargetPosL=Trajectory(1:3,CurrentState)+0.27*[0;cos(Trajectory(4,CurrentState)/180*pi);sin(Trajectory(4,CurrentState)/180*pi)];
    DesiredJointStatesR=GenInvKinR(PreviousMeasureR,TargetPosR,rotx(90+Trajectory(4,CurrentState)),JointBounds2);
    DesiredJointStatesL=GenInvKinL(PreviousMeasureL,TargetPosL,rotx(90+Trajectory(4,CurrentState)),JointBounds2);
    entry,during:
    GripCommand=1;
    PosDiffR=eePoseR-TargetPosR;
    PosDiffL=eePoseL-TargetPosL;
    AngleRef=Trajectory(4,CurrentState);
  state PREP_ROTATION
    entry:
    ReachedState=3;
    DesiredJointStatesR=[pi/6;0;pi/2;pi/2;-pi/2;0;pi/2];
    DesiredJointStatesL=DesiredJointStatesR;
    entry,during:
    GripCommand=1;
    PosDiffR=eePoseR-TargetPosR;
    PosDiffL=eePoseL-TargetPosL;
  state CHECK_TOLERANCE
    entry,during:
    GripCommand=1;
    PosDiffR=eePoseR-TargetPosR;
    PosDiffL=eePoseL-TargetPosL;
  DETECTION_AND_OBJECT_APPROACH -> GRABBING : [checkTolerance]
  GRABBING -> WAIT_GRABBING : after(0.5,sec)
  (default) -> DETECTION_AND_OBJECT_APPROACH : {CurrentState=1}
  DELAY_CHECKING -> ENDING [order 3] : [checkTolerance&&detectObject&&ReachedState==size(Trajectory,2)+3]
  WAIT_GRABBING -> DETECTION_AND_OBJECT_APPROACH [order 1] : [~detectObject]
      | {GripCommand=0}
  DELAY_CHECKING -> DETECTION_AND_OBJECT_APPROACH [order 1] : [~detectObject]
      | {GripCommand=0}
  SET_CONFIG -> DETECTION_AND_OBJECT_APPROACH [order 1] : [~detectObject]
      | {GripCommand=0}
  PREP_ROTATION -> DETECTION_AND_OBJECT_APPROACH [order 1] : [~detectObject]
      | {GripCommand=0}
  WAIT_GRABBING -> PREP_ROTATION [order 2] : [detectObject]
  DELAY_CHECKING -> SET_CONFIG [order 4] : [checkTolerance&&detectObject]
  CHECK_TOLERANCE -> DELAY_CHECKING : after(0.2,sec)
  DELAY_CHECKING -> CHECK_TOLERANCE [order 2] : [~checkTolerance]
  PREP_ROTATION -> SET_CONFIG [order 2] : [detectObject]
      | {CurrentState=0}
  SET_CONFIG -> CHECK_TOLERANCE [order 2] : [checkTolerance&&detectObject]
  data: isBall function_output; previousConfig function_input; eePosition function_input; jointStatesL function_output; rotMatrix function_input; JointBoundaries function_input; previousConfig function_input; eePosition function_input; jointStatesR function_output; rotMatrix function_input; JointBoundaries function_input; atState function_output; Trajectory input; eeTolerance input; angleTolerance input; rotM1 input; TargetPosR local; JointBounds1 input; JointBounds2 input; PreviousMeasureR input; PreviousMeasureL input; ObjectPosition input; eePoseR input; eePoseL input; GripForceR input; GripForceL input; TargetPosL local; ReachedState output; DesiredJointStatesR output; DesiredJointStatesL output; GripCommand output; CurrentState local; PosDiffR output; PosDiffL output; AngleRef output; ObjectAngle input
  function isBall = detectObject:
    | function isBall = detectObject
    | %% Checks the presence of a ball in RIGHT HAND based on a minimum force threshold
    | isBallR = all(abs(GripForceR)>7);
    | %% Checks the presence of a ball in LEFT HAND based on a minimum force threshold
    | isBallL = all(abs(GripForceL)>7);
    | 
    | isBall = isBallR && isBallL;
  function jointStatesL = GenInvKinL(previousConfig,eePosition,rotMatrix,JointBoundaries):
    | function jointStatesL = GenInvKinL(previousConfig,eePosition,rotMatrix,JointBoundaries)
    | coder.extrinsic('IKL')
    | jointStatesL=zeros(7,1);
    | jointStatesL=IKL(eePosition,previousConfig,rotMatrix,JointBoundaries);
  function jointStatesR = GenInvKinR(previousConfig,eePosition,rotMatrix,JointBoundaries):
    | function jointStatesR = GenInvKinR(previousConfig,eePosition,rotMatrix,JointBoundaries)
    | coder.extrinsic('IKR')
    | jointStatesR=zeros(7,1);
    | jointStatesR=IKR(eePosition,previousConfig,rotMatrix,JointBoundaries);
  function atState = checkTolerance:
    | function atState = checkTolerance
    | 
    | % Check if a robot state RIGHT has been reached within tolerance
    | reachedPointR = all(abs(eePoseR-TargetPosR) < eeTolerance);
    | % Check if a robot state LEFT has been reached within tolerance
    | reachedPointL = all(abs(eePoseL-TargetPosL) < eeTolerance);
    | % Check if a robot ANGLE has been reached within tolerance
    | reachedAngle = (abs(ObjectAngle-AngleRef) < angleTolerance);
    | 
    | atState = reachedPointR && reachedPointL && reachedAngle;
